simulink model "LQI_controller"  (R2025b)
settings: Solver=VariableStepAuto  StartTime=0.0  StopTime=10.0  RelTol=1e-3
undefined symbols (not defined in the file): alpha, DiscIntNeverNeededParam, dspblkCoreblockFVToolHelper, gcbh, K1, K2, K3, Ts
settings Model: Creator=samue  LastModifiedBy=samue

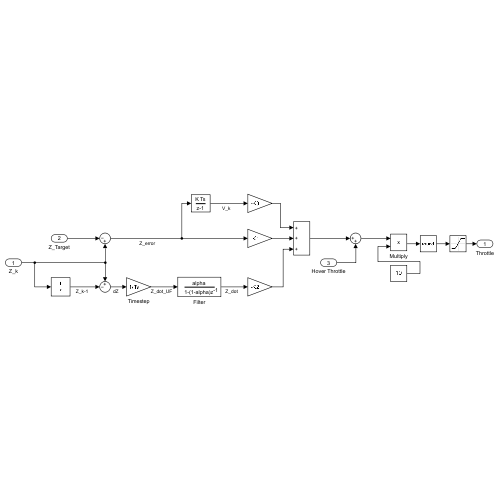
[thumbnail: Simulink's stored preview of the top-level diagram]
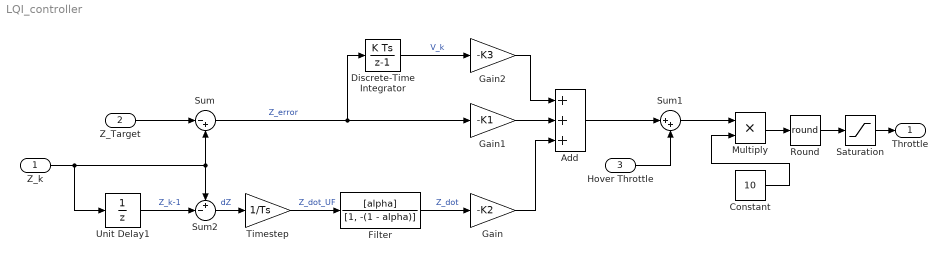
== system LQI_controller ==
  Z_k : Inport
  Z_Target : Inport  Port=2
  Hover Throttle : Inport  Port=3
  Add : Sum  Inputs=+++
  Constant : Constant  Value=10
  Discrete-Time Integrator : DiscreteIntegrator  SampleTime=-1  ICPrevOutput=DiscIntNeverNeededParam  ICPrevScaledInput=DiscIntNeverNeededParam
  Filter : DiscreteFilter  LoadFcn=dspblkCoreblockFVToolHelper(gcbh,'load');  Numerator=[alpha]  Denominator=[1, -(1 - alpha)]
      settings: CopyFcn=dspblkCoreblockFVToolHelper(gcbh,'copy');  DeleteFcn=dspblkCoreblockFVToolHelper(gcbh,'close');  ModelCloseFcn=dspblkCoreblockFVToolHelper(gcbh,'close');  PreSaveFcn=dspblkCoreblockFVToolHelper(gcbh,'presave');  PostSaveFcn=dspblkCoreblockFVToolHelper(gcbh,'postsave');  CloseFcn=dspblkCoreblockFVToolHelper(gcbh,'close');
  Gain : Gain  Gain=-K2
  Gain1 : Gain  Gain=-K1
  Gain2 : Gain  Gain=-K3
  Multiply : Product
  Round : Rounding  Operator=round
  Saturation : Saturate  UpperLimit=1000  LowerLimit=0
  Sum : Sum  Inputs=|-+
  Sum1 : Sum  Inputs=|++
  Sum2 : Sum  Inputs=+-|
  Timestep : Gain  Gain=1/Ts
  Unit Delay1 : UnitDelay  SampleTime=-1  StateName=Z  HasFrameUpgradeWarning=on
  "Throttle " : Outport  VectorParamsAs1DForOutWhenUnconnected=off
  wires:
  Z_k/1 -> Sum2/1, Sum/2, Unit Delay1/1
  Round/1 -> Saturation/1
  Constant/1 -> Multiply/2
  Add/1 -> Sum1/1
  Hover Throttle/1 -> Sum1/2
  Multiply/1 -> Round/1
  Z_Target/1 -> Sum/1
  Sum1/1 -> Multiply/1
  Saturation/1 -> "Throttle "/1
  Sum/1 -> Gain1/1, Discrete-Time Integrator/1  "Z_error"
  Gain1/1 -> Add/2
  Gain/1 -> Add/3
  Sum2/1 -> Timestep/1  "dZ"
  Timestep/1 -> Filter/1  "Z_dot_UF"
  Gain2/1 -> Add/1
  Unit Delay1/1 -> Sum2/2  "Z_k-1"
  Discrete-Time Integrator/1 -> Gain2/1  "V_k"
  Filter/1 -> Gain/1  "Z_dot"
